simulink model "kf_discrete_time"  (R2018b)
settings: Solver=FixedStepAuto  StartTime=0.0  StopTime=15  FixedStep=1e-3  RelTol=1e-3
values from neighbouring files (symbols this model uses):
  A = obj.A    [LeftLaneChangeRelativeMotionModel.m]    (also in initialization.m = 1.75; laneChangeSinusoidalFcn.m = 1.75; laneChangeSinusoidalJacobianFcn.m = 1.75; leftLaneChangeParametricFcn.m = lateral_dist/2)
  Ts = 0.1    [KinematicBicycleModel.m]    (also in LeftLaneChangeSinusoidalMotionModel.m; LinearizedBicycleModel.m; SimplifiedKinematicBicycleModel.m; amm_rel_test.m)
  vx = X(2)    [cv_model_fun.m]    (also in initialization.m = 10)
  vy = X(4)    [cv_model_fun.m]    (also in initialization.m = 0)
  w = obj.w    [LeftLaneChangeRelativeMotionModel.m]    (also in ctra_model_fun.m = X(6); ctrv_model_fun.m = X(5); initialization.m = 0.0314159265359; laneChangeSinusoidalFcn.m = 0.0209439510239)
  x = X(1)    [KinematicBicycleModel.m]    (also in SimplifiedKinematicBicycleModel.m; behavior_model.m = 0:0.01:20; cca_model_fun.m; ctra_model_fun.m)
  y = X(2)    [KinematicBicycleModel.m]    (also in SimplifiedKinematicBicycleModel.m; behavior_model.m = [distances velocities]; cca_model_fun.m; ctra_model_fun.m)
  y_init = lanewidth/2    (= 1.75)    [initialization.m]    (also in laneChangeSinusoidalFcn.m; laneChangeSinusoidalJacobianFcn.m; leftLaneChangeSinusoidalFcn.m; leftLaneChangeSinusoidalJacobianFcn.m)
undefined symbols (not defined in the file or in its folder): Discrete, Time
libraries: simulink x5, sharedTrackingLibrary x2, ctrlSharedLib x1, dspadpt3 x1
settings Model: Creator=jasprit  LastModifiedBy=jasprit
settings SFSimCC: SimUseLocalCustomCode=off
settings RTWCC: RTWUseLocalCustomCode=off

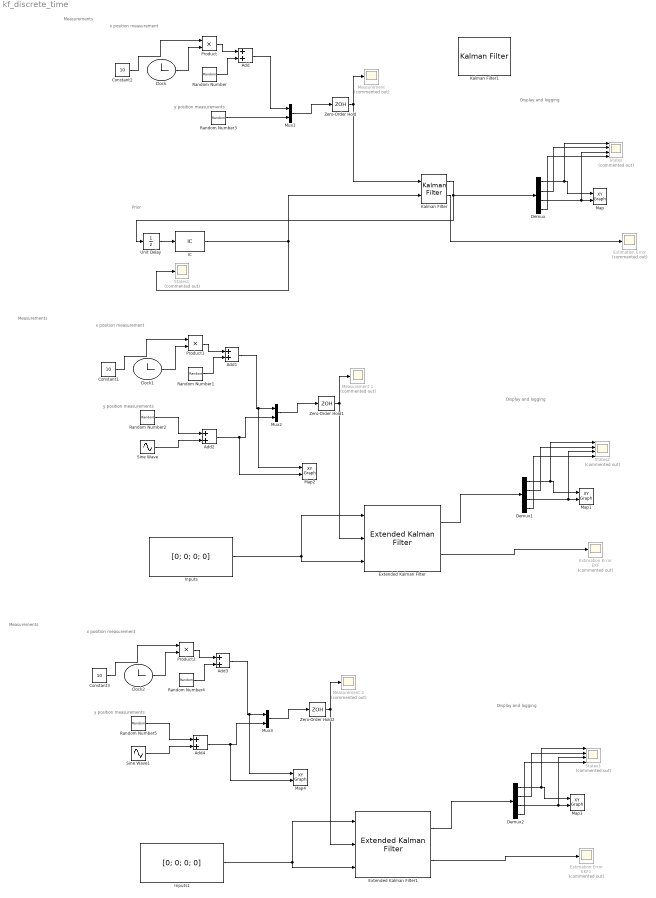
== system kf_discrete_time ==
  note: y position measurements
  note: x position measurement
  note: Display and logging
  note: Prior
  note: Measurements
  note: x position measurement
  note: Display and logging
  note: Measurements
  note: y position measurements
  note: y position measurements
  note: Measurements
  note: Display and logging
  note: x position measurement
  Add{,1..4} (5 alike) : Sum
  Clock : Clock
  Clock1 : Clock
  Clock2 : Clock
  Constant1 : Constant  Value=10
  Constant2 : Constant  Value=10
  Constant3 : Constant  Value=10
  Demux : Demux
  Demux1 : Demux
  Demux2 : Demux
  Estimation Error : Scope  Commented=on
  Estimation Error EKF : Scope  Commented=on
  Estimation Error EKF1 : Scope  Commented=on
  Extended Kalman Filter : sharedTrackingLibrary/Extended Kalman Filter  StateTransitionFcn=laneChangeSinusoidalFcn  HasStateTransitionJacobianFcn=on  StateTransitionJacobianFcn=laneChangeSinusoidalJacobianFcn  HasAdditiveProcessNoise=Additive  ProcessNoise=[0.5 5 0.5 5]'  HasTimeVaryingProcessNoise=off  HasStateTransitionFcnExtraArgument=1  InitialState=[0 10 0 0]  InitialStateCovariance=1e-6  MeasurementFcn1=positionMeasurementFcn  HasMeasurementJacobianFcn1=off  HasMeasurementEnablePort1=off  HasAdditiveMeasurementNoise1=Additive  MeasurementNoise1=[0.2 0; 0 0.2]  HasTimeVaryingMeasurementNoise1=off  HasMeasurementFcnExtraArgument1=1  MeasurementFcn2=myMeasurementFcn  HasMeasurementJacobianFcn2=off  HasMeasurementEnablePort2=off  HasAdditiveMeasurementNoise2=Additive  MeasurementNoise2=1  HasTimeVaryingMeasurementNoise2=off  HasMeasurementFcnExtraArgument2=0  MeasurementFcn3=myMeasurementFcn  HasMeasurementJacobianFcn3=off  HasMeasurementEnablePort3=off  HasAdditiveMeasurementNoise3=Additive  MeasurementNoise3=1  HasTimeVaryingMeasurementNoise3=off  HasMeasurementFcnExtraArgument3=0  MeasurementFcn4=myMeasurementFcn  HasMeasurementJacobianFcn4=off  HasMeasurementEnablePort4=off  HasAdditiveMeasurementNoise4=Additive  MeasurementNoise4=1  HasTimeVaryingMeasurementNoise4=off  HasMeasurementFcnExtraArgument4=0  MeasurementFcn5=myMeasurementFcn  HasMeasurementJacobianFcn5=off  HasMeasurementEnablePort5=off  HasAdditiveMeasurementNoise5=Additive  MeasurementNoise5=1  HasTimeVaryingMeasurementNoise5=off  HasMeasurementFcnExtraArgument5=0  EnableMultirate=off  StateTransitionFcnSampleTime=1  MeasurementFcn1SampleTime=1  MeasurementFcn2SampleTime=1  MeasurementFcn3SampleTime=1  MeasurementFcn4SampleTime=1  MeasurementFcn5SampleTime=1  UseCurrentEstimator=on  OutputStateCovariance=on  DataType=double  SampleTime=Ts  NumberOfMeasurements=1
      settings: SourceProductName=Control System Toolbox  SourceProductBaseCode=CT
  Extended Kalman Filter1 : sharedTrackingLibrary/Extended Kalman Filter  StateTransitionFcn=leftLaneChangeSinusoidalFcn  HasStateTransitionJacobianFcn=on  StateTransitionJacobianFcn=leftLaneChangeSinusoidalJacobianFcn  HasAdditiveProcessNoise=Additive  ProcessNoise=[0.5 5 0.5 5]'  HasTimeVaryingProcessNoise=off  HasStateTransitionFcnExtraArgument=1  InitialState=[0 10 0 0]  InitialStateCovariance=1e-6  MeasurementFcn1=positionMeasurementFcn  HasMeasurementJacobianFcn1=off  HasMeasurementEnablePort1=off  HasAdditiveMeasurementNoise1=Additive  MeasurementNoise1=[0.2 0; 0 0.2]  HasTimeVaryingMeasurementNoise1=off  HasMeasurementFcnExtraArgument1=1  MeasurementFcn2=myMeasurementFcn  HasMeasurementJacobianFcn2=off  HasMeasurementEnablePort2=off  HasAdditiveMeasurementNoise2=Additive  MeasurementNoise2=1  HasTimeVaryingMeasurementNoise2=off  HasMeasurementFcnExtraArgument2=0  MeasurementFcn3=myMeasurementFcn  HasMeasurementJacobianFcn3=off  HasMeasurementEnablePort3=off  HasAdditiveMeasurementNoise3=Additive  MeasurementNoise3=1  HasTimeVaryingMeasurementNoise3=off  HasMeasurementFcnExtraArgument3=0  MeasurementFcn4=myMeasurementFcn  HasMeasurementJacobianFcn4=off  HasMeasurementEnablePort4=off  HasAdditiveMeasurementNoise4=Additive  MeasurementNoise4=1  HasTimeVaryingMeasurementNoise4=off  HasMeasurementFcnExtraArgument4=0  MeasurementFcn5=myMeasurementFcn  HasMeasurementJacobianFcn5=off  HasMeasurementEnablePort5=off  HasAdditiveMeasurementNoise5=Additive  MeasurementNoise5=1  HasTimeVaryingMeasurementNoise5=off  HasMeasurementFcnExtraArgument5=0  EnableMultirate=off  StateTransitionFcnSampleTime=1  MeasurementFcn1SampleTime=1  MeasurementFcn2SampleTime=1  MeasurementFcn3SampleTime=1  MeasurementFcn4SampleTime=1  MeasurementFcn5SampleTime=1  UseCurrentEstimator=on  OutputStateCovariance=on  DataType=double  SampleTime=Ts  NumberOfMeasurements=1
      settings: SourceProductName=Control System Toolbox  SourceProductBaseCode=CT
  IC : InitialCondition  Value=[x vx y vy]
  Inputs : Constant  Value=[0; 0; 0; 0]  SampleTime=Ts
  Inputs1 : Constant  Value=[0; 0; 0; 0]  SampleTime=Ts
  Kalman Filter : ctrlSharedLib/Kalman Filter  TimeDomain=Discrete-Time  UseCurrentEstimator=on  ModelSource=Individual A, B, C, D matrices  ModelSourceVariable=ss(0.95,1,1,0,1)  A=[1 Ts 0 0; 0 1 0 0; 0 0 1 Ts; 0 0 0 1]  B=[1 0; 0 1]  C=[1 0 0 0; 0 0 1 0]  D=[0 0; 0 0]  NumberOfStates=1  NumberOfInputs=1  NumberOfOutputs=1  InitialEstimateSource=Input port  X0=[0 0 20 0]  P0=10  UseK=off  UseGH=off  NumberOfProcessNoiseInputs=1  G=1  TimeInvariantG=on  H=0  TimeInvariantH=on  Q=[0.5 5 0.5 5]'  TimeInvariantQ=on  R=[0.2 0; 0 0.2]  TimeInvariantR=on  N=0  TimeInvariantN=on  AddInputPort=off  AddEnablePort=off  OutputEstimatedY=off  OutputP=on  Ts=Ts
      settings: SourceProductBaseCode=CT
  Kalman Filter1 : dspadpt3/Kalman Filter  num_targets=10  sourceEnable=Specify via input port <Enable>  isReset=on  X=zeros([6, 1])  P=10*eye(6)  A=[1 0 1 0 0 0;0 1 0 1 0 0; 0 0 1 0 0 0; 0 0 0 1 0 0; 0 0 0 0 1 0; 0 0 0 0 0 1]  sourceMeasure=Specify via Dialog  H=[1 0 0 0 0 0; 0 1 0 0 0 0; 0 0 0 0 1 0; 0 0 0 0 0 1]  Q=0.05*eye(6)  R=eye(4)  isOutputEstMeasure=on  isOutputEstState=off  isOutputEstError=off  isOutputPrdMeasure=off  isOutputPrdState=off  isOutputPrdError=off
      settings: SourceProductName=DSP System Toolbox  SourceProductBaseCode=DS
  Map : simulink/Sinks/XY Graph  xmin=-1  xmax=200  ymin=-20  ymax=20  st=-1
  Map{1..4} (4 alike) : simulink/Sinks/XY Graph  xmin=-1  xmax=200  ymin=-5  ymax=5  st=-1
  "Measurement " : Scope  Commented=on
  Measurement 1 : Scope  Commented=on
  Measurement 2 : Scope  Commented=on
  Mux1 : Mux  Inputs=2
  Mux2 : Mux  Inputs=2
  Mux3 : Mux  Inputs=2
  Product : Product
  Product1 : Product
  Product2 : Product
  Random Number : RandomNumber  Variance=0.1  SampleTime=Ts
  Random Number1 : RandomNumber  Variance=0.1  SampleTime=Ts
  Random Number2 : RandomNumber  Variance=0.2  SampleTime=Ts
  Random Number3 : RandomNumber  Variance=0.2  SampleTime=Ts
  Random Number4 : RandomNumber  Variance=0.1  SampleTime=Ts
  Random Number5 : RandomNumber  Variance=0.2  SampleTime=Ts
  Sine Wave : Sin  Amplitude=A  Bias=-A  Frequency=w*vx  Phase=+pi/2  SampleTime=Ts
  Sine Wave1 : Sin  Amplitude=A  Bias=y_init  Frequency=w*vx  Phase=-pi/2  SampleTime=Ts
  States : Scope  Commented=on  NumInputPorts=4
  States1 : Scope  Commented=on
  States2 : Scope  Commented=on  NumInputPorts=4
  States3 : Scope  Commented=on  NumInputPorts=4
  Unit Delay : UnitDelay  SampleTime=-1
  Zero-Order Hold : ZeroOrderHold  SampleTime=Ts
  Zero-Order Hold1 : ZeroOrderHold  SampleTime=Ts
  Zero-Order Hold2 : ZeroOrderHold  SampleTime=Ts
  wires:
  Constant2/1 -> Product/1
  Kalman Filter/1 -> Unit Delay/1, Demux/1
  Demux/1 -> States/1, Map/1
  Clock/1 -> Product/2
  Product/1 -> Add/1
  Random Number/1 -> Add/2
  Add/1 -> Mux1/1
  Kalman Filter/2 -> Estimation Error/1
  Demux/2 -> States/2
  Mux1/1 -> Zero-Order Hold/1
  Random Number3/1 -> Mux1/2
  Demux/3 -> Map/2, States/3
  Demux/4 -> States/4
  IC/1 -> States1/1, Kalman Filter/2
  Zero-Order Hold/1 -> Kalman Filter/1, "Measurement "/1
  Unit Delay/1 -> IC/1
  Zero-Order Hold1/1 -> Extended Kalman Filter/2, Measurement 1/1
  Extended Kalman Filter/1 -> Demux1/1
  Demux1/4 -> States2/4
  Demux1/1 -> States2/1, Map1/1
  Product1/1 -> Add1/1
  Clock1/1 -> Product1/2
  Constant1/1 -> Product1/1
  Demux1/2 -> States2/2
  Mux2/1 -> Zero-Order Hold1/1
  Add1/1 -> Map2/1, Mux2/1
  Demux1/3 -> Map1/2, States2/3
  Random Number1/1 -> Add1/2
  Random Number2/1 -> Add2/1
  Sine Wave/1 -> Add2/2
  Add2/1 -> Map2/2, Mux2/2
  Inputs/1 -> Extended Kalman Filter/3, Extended Kalman Filter/1
  Extended Kalman Filter/2 -> Estimation Error EKF/1
  Random Number5/1 -> Add4/1
  Add3/1 -> Map4/1, Mux3/1
  Clock2/1 -> Product2/2
  Sine Wave1/1 -> Add4/2
  Extended Kalman Filter1/1 -> Demux2/1
  Product2/1 -> Add3/1
  Demux2/2 -> States3/2
  Random Number4/1 -> Add3/2
  Constant3/1 -> Product2/1
  Extended Kalman Filter1/2 -> Estimation Error EKF1/1
  Mux3/1 -> Zero-Order Hold2/1
  Demux2/4 -> States3/4
  Demux2/3 -> Map3/2, States3/3
  Demux2/1 -> States3/1, Map3/1
  Add4/1 -> Map4/2, Mux3/2
  Zero-Order Hold2/1 -> Extended Kalman Filter1/2, Measurement 2/1
  Inputs1/1 -> Extended Kalman Filter1/3, Extended Kalman Filter1/1
